simulink model "pos_test"  (R2019a)
settings: Solver=FixedStepAuto  StartTime=0.0  StopTime=10.0  RelTol=1e-3  EnableMultiTasking=on
values from neighbouring files (symbols this model uses):
  ts = 1/50    (= 0.02)    [sim_init.m]    (also in sim_param.mat; velo_id_tc.m; velo_pi_mdb.m)
libraries: arduinolib x3
settings Model: ExtModeTrigDuration=2  Creator=Daichi  LastModifiedBy=Daichi
settings OptimizationCC: EnhancedBackFolding=on  PassReuseOutputArgsAs=Individual arguments  MaxStackSize=64  OptimizeBlockOrder=speed  DifferentSizesBufferReuse=on  OptimizationCustomize=off
settings DebuggingCC: ParameterTunabilityLossMsg=error
settings HardwareCC: ProdBitPerInt=16  ProdBitPerPointer=16  ProdBitPerSizeT=16  ProdBitPerPtrDiffT=16  ProdLargestAtomicFloat=None  ProdWordSize=8  ProdHWDeviceType=Atmel->AVR  UseEmbeddedCoderFeatures=off
settings SFSimCC: MATLABDynamicMemAlloc=off
settings RTWCC: SystemTargetFile=ert.tlc  HardwareBoard=Arduino Mega 2560  TLCOptions=-aInlineSetEventsForThisBaseRateFcn=TLC_FALSE -aSuppressMultiTaskScheduler=TLC_FALSE -aRateBasedStepFcn=1  TemplateMakefile=ert_default_tmf  GenerateReport=on  Toolchain=Arduino AVR  BuildConfiguration=Faster Runs  IncludeHyperlinkInReport=on  LaunchReport=on  GenerateTraceInfo=on  GenerateTraceReport=on  GenerateTraceReportSl=on  GenerateTraceReportSf=on  GenerateTraceReportEml=on
settings CodeAppCC: ForceParamTrailComments=on  IgnoreCustomStorageClasses=off  OperatorAnnotations=on  SimulinkDataObjDesc=on  SFDataObjDesc=on  InsertBlockDesc=on
settings ERTTargetCC: SupportContinuousTime=on  SupportNonInlinedSFcns=on  SupportVariableSizeSignals=on  ExtModeStaticAllocSize=2048

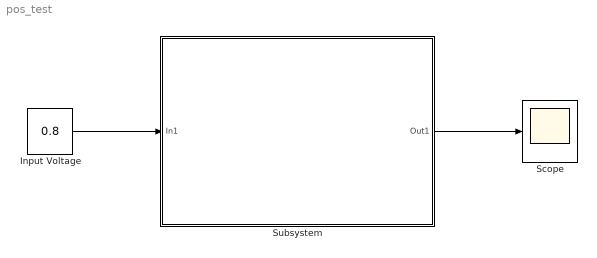
== system pos_test ==
  "Input Voltage " : Constant  Value=0.8
  Scope : Scope
  Subsystem : Subsystem
  wires:
  "Input Voltage "/1 -> Subsystem/1(In1)
  Subsystem/1(Out1) -> Scope/1

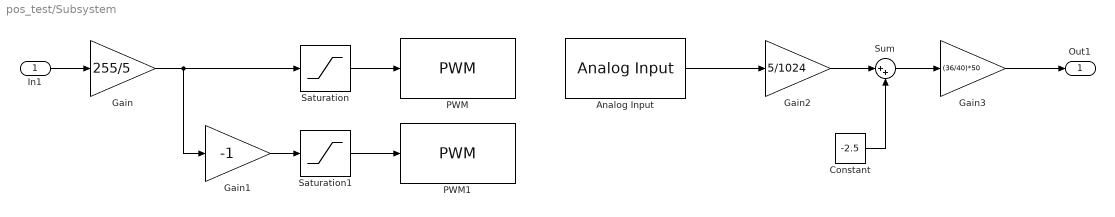
== system pos_test/Subsystem ==
  In1 : Inport
  Analog Input : arduinolib/Analog Input  pinNumber=0  ReadResultsOnly=off  ConversionTriggerSource=Software  ExternalTriggerType=uint32(0)  OutputDataType=uint16  EnableConversionCompleteNotify=off  EnableOuputStatus=off  SampleTime=ts  blockPlatform=arduino
  Constant : Constant  Value=-2.5
  Gain : Gain  Gain=255/5
  Gain1 : Gain  Gain=-1
  Gain2 : Gain  Gain=5/1024
  Gain3 : Gain  Gain=(36/40)*50
  PWM : arduinolib/PWM  pinNumber=3  EnableInputFrequency=off  InitialFrequency=2000  InitialDutyCycle=0  NotificationType=None  blockPlatform=arduino
  PWM1 : arduinolib/PWM  pinNumber=5  EnableInputFrequency=off  InitialFrequency=2000  InitialDutyCycle=0  NotificationType=None  blockPlatform=arduino
  Saturation : Saturate  UpperLimit=255  LowerLimit=0
  Saturation1 : Saturate  UpperLimit=255  LowerLimit=0
  Sum : Sum  Inputs=|++
  Out1 : Outport
  wires:
  Gain/1 -> Gain1/1, Saturation/1
  In1/1 -> Gain/1
  Sum/1 -> Gain3/1
  Gain2/1 -> Sum/1
  Gain1/1 -> Saturation1/1
  Constant/1 -> Sum/2
  Analog Input/1 -> Gain2/1
  Gain3/1 -> Out1/1
  Saturation/1 -> PWM/1
  Saturation1/1 -> PWM1/1
